simulink model "dumbSystem"  (R2020b)
settings: Solver=VariableStepAuto  StartTime=0.0  StopTime=20  RelTol=1e-3
values from neighbouring files (symbols this model uses):
  basin1 = 55560000    [data.mat]
  k = 1    [data.mat]
  n = 0.02    [data.mat]
  R = 0.75    [data.mat]
  S = 0.2    [data.mat]
undefined symbols (not defined in the file or in its folder): C, d
settings Model: Creator=valstandard  LastModifiedBy=valstandard

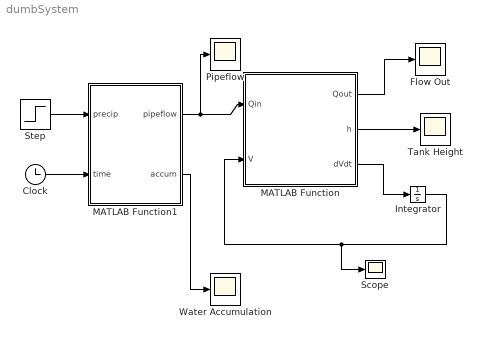
== system dumbSystem ==
  " Pipeflow" : Scope
  Clock : Clock
  Flow Out : Scope
  Integrator : Integrator  InitialCondition=70
  MATLAB Function : MATLAB Function  TreatAsAtomicUnit=on
  MATLAB Function1 : MATLAB Function  TreatAsAtomicUnit=on
  Scope : Scope
  Step : Step  Time=5  After=0.002  SampleTime=0
  Tank Height : Scope
  Water Accumulation : Scope
  wires:
  Step/1 -> MATLAB Function1/1(precip)
  MATLAB Function/3(dVdt) -> Integrator/1
  Integrator/1 -> MATLAB Function/2(V), Scope/1
  MATLAB Function/1(Qout) -> Flow Out/1
  MATLAB Function/2(h) -> Tank Height/1
  MATLAB Function1/1(pipeflow) -> " Pipeflow"/1, MATLAB Function/1(Qin)
  MATLAB Function1/2(accum) -> Water Accumulation/1
  Clock/1 -> MATLAB Function1/2(time)

== matlab function dumbSystem/MATLAB Function1 ==
  data: pipeflow output; precip input; k parameter; n parameter; R parameter; S parameter; basin1 parameter; time input; accum output
function [pipeflow, accum]  = pipeflow(precip, k, n, R, S, basin1, time)
% v = k*n*R^0.63*S^.54
% cross sectional area: pi*r^2
% v = velocity; n = roughness; R = hydraulic radius; S = slope; k =
% conversions

v = k*n*R^0.63*S^.54; %should be 
Ax = pi*R^2;
pipeflowMax = v*Ax; %pipe flow out is 4.82 m3/s
% if water coming in is below max, it flows in normally
% if above max, then it flows according to the max flow
if precip*basin1 < pipeflowMax
    pipeflow = precip*basin1
else
    pipeflow = pipeflowMax
end
accum = precip*basin1*time - pipeflow*time;
% h = precip*clock; %calculates the accumulated precipitation
% Qout = C*sqrt(h); 
% dPdt = pipeflow - Qout; %change in volume; 
% % where if dVdt > volume of tank, there's a back up in system
% 
% % dPdt = basin1*precip + wateracc - pipeflow; %water remaining to be assimilated

== matlab function dumbSystem/MATLAB Function ==
  data: Qout output; h output; Qin input; dVdt output; V input; d parameter; C parameter
function [Qout, h, dVdt] = tank(Qin, V, d, C)
% Qin = flow rate in in inches per time
% V = volume
% Ax = cross sectional area

%%%%%% MY code%%%%%%
% Qinm = Qin*1.63871*10^(-5); %convert to m^3 per time
% h = V/Ax; %height of water in tank
% Qout = C*sqrt(h); %water flowing out m^3/time

%%%%%%% copied code %%%%%%
Axs = pi/4*d^2;
h = V/Axs;
Qout = C*sqrt(h);
dVdt = Qin - Qout; %change in volume; 
% where if dVdt > volume of tank, there's a back up in system
